simulink model "VSM_specComp_DC_22a"  (R2022a)
settings: Solver=ode3  StartTime=0.0  StopTime=4  FixedStep=HWSampleTime  RelTol=1e-3
PostLoadFcn:
  | EXEC_MODE=ExecutionMode.SIMULATION;
  | %Sim_TP33_VSM_HSS_init
InitFcn:
  | %EXEC_MODE=ExecutionMode.SIMULATION;
  | %Sim_TP33_VSM_HSS_init
StopFcn:
  | %sim2struct
undefined symbols (not defined in the file): ControlSampleTime, DiscIntNeverNeededParam, fault_dur, Grid, HWSampleTime, Ion, LCL, Lithium, Manage, Param, SM, t_fault, V_DC, VSMCTRL
libraries: FriedrichLibrary x76, simulink x32, TriphaseHardwaremodule x24, spsThreePhaseSeriesRLCBranchLib x8, spsThreePhaseVIMeasurementLib x8, spsThreePhaseBreakerLib x8, spsGroundLib x4, spsUniversalBridgeLib x4, spsVoltageMeasurementLib x4, spsEdgeDetectorLib x4, spsMeanLib x4, simulink_extras x4
(part 7 of 10)

== system VSM_specComp_DC_22a/VSM_1/VSM1/VSM/CONTROL/Virtual Circuit1/PT1 ==
  U : Inport  SampleTime=Ts
  tau : Inport  Port=2  SampleTime=Ts
  Reset : Inport  Port=3  SampleTime=Ts
  Delay : Delay  DelayLength=1
  Divide : Product  Inputs=*/
  Gain : Gain  Gain=Ts
  Gain1 : Gain  Gain=K
  Saturation : Saturate  UpperLimit=inf  LowerLimit=Ts
  Sum : Sum  Inputs=|++
  Sum2 : Sum  Inputs=|+-
  Switch : Switch  Criteria=u2 > Threshold  SaturateOnIntegerOverflow=off  InputSameDT=off
  Y : Outport
  wires:
  Reset/1 -> Switch/2
  Saturation/1 -> Divide/2
  Divide/1 -> Sum/1
  tau/1 -> Saturation/1
  Delay/1 -> Sum2/2, Sum/2
  Gain/1 -> Divide/1
  U/1 -> Switch/1, Sum2/1
  Sum2/1 -> Gain/1
  Gain1/1 -> Y/1
  Switch/1 -> Gain1/1, Delay/1
  Sum/1 -> Switch/3

== system VSM_specComp_DC_22a/VSM_1/VSM1/VSM/CONTROL/Virtual Circuit1/PT2 ==
  U : Inport  SampleTime=Ts
  tau : Inport  Port=2  SampleTime=Ts
  Reset : Inport  Port=3  SampleTime=Ts
  Phi : Inport  Port=4
  Delay : Delay  DelayLength=1  InitialConditionSource=Input port  ExternalReset=Rising
      settings: InputPortMap=u0,r5,p4
  Divide : Product  Inputs=*/
  Gain : Gain  Gain=Ts
  Gain1 : Gain  Gain=K
  Saturation : Saturate  UpperLimit=inf  LowerLimit=Ts
  Sum : Sum  Inputs=|++
  Sum2 : Sum  Inputs=|+-
  Unit Delay2 : UnitDelay  InitialCondition=[0 0 0]  SampleTime=ControlSampleTime  HasFrameUpgradeWarning=on
  dq0->ab0 phi1 : FriedrichLibrary/Transformations/dq0->ab0 phi  SystemSampleTime=-1  VariantActivationTime=update diagram  Latency=0  AutoFrameSizeCalculation=off
  Y : Outport
  wires:
  dq0->ab0 phi1/1 -> Delay/3
  Gain1/1 -> Y/1
  Sum2/1 -> Gain/1
  U/1 -> Sum2/1
  Gain/1 -> Divide/1
  Delay/1 -> Sum/2, Sum2/2
  tau/1 -> Saturation/1
  Divide/1 -> Sum/1
  Saturation/1 -> Divide/2
  Reset/1 -> Delay/2
  Sum/1 -> Delay/1, Unit Delay2/1, Gain1/1
  Unit Delay2/1 -> dq0->ab0 phi1/1
  Phi/1 -> dq0->ab0 phi1/2

== system VSM_specComp_DC_22a/VSM_1/VSM1/VSM/CONTROL/i_dq_ctrl/PI ==
  di : Inport
  u0 : Inport  Port=2
  Enable : EnablePort  StatesWhenEnabling=reset
  Gain4 : Gain  Gain=Ki
  Gain5 : Gain  Gain=Kp
  Integrator (inertia) : DiscreteIntegrator  gainval=1  InitialConditionSource=external  InitialCondition=1  SampleTime=ControlSampleTime  ICPrevOutput=DiscIntNeverNeededParam  ICPrevScaledInput=DiscIntNeverNeededParam
  Product : Product
  Product1 : Product
  Step : Step  Time=8  Before=1  SampleTime=0
  Step1 : Step  Time=8.05+10  Before=1  After=0.1  SampleTime=0
  Sum2 : Sum  Inputs=++|
  u : Outport  VectorParamsAs1DForOutWhenUnconnected=off
  wires:
  u0/1 -> Integrator (inertia)/2
  Sum2/1 -> u/1
  di/1 -> Gain4/1, Gain5/1
  Integrator (inertia)/1 -> Sum2/2
  Gain5/1 -> Product/2
  Gain4/1 -> Product1/2
  Product1/1 -> Integrator (inertia)/1
  Product/1 -> Sum2/1
  Step/1 -> Product/1
  Step1/1 -> Product1/1

== system VSM_specComp_DC_22a/VSM_1/VSM1/VSM/MANAGEMENT/Subsystem1/Subsystem ==
  note: zweiter Faktor bei clearing für richtiges Q
      |
      | bei Eintritt mit Halten aber fester Grenze
      |
      | bis jetzt über Zeit abgeschaltet bei clearing ohne Halten
  i_inv : Inport
  PQ_out : Inport  Port=2
  iabs : Inport  Port=3
  U_cap : Inport  Port=4
  PQ_pre : Inport  Port=5
  i abs_pre : Inport  Port=6
  Enable : EnablePort
  Abs : Abs  SaturateOnIntegerOverflow=off
  Add : Sum  Inputs=+-
  Demux : Demux  Commented=on  Outputs=3
  Discrete Derivative1 : simulink/Discrete/Discrete Derivative  Commented=on  gainval=1.0  ICPrevScaledInput=0.0  OutMin=[]  OutMax=[]  OutDataType=fixdt(1, 16)  OutScaling=2^-10  DoSatur=off
  Discrete Derivative2 : simulink/Discrete/Discrete Derivative  gainval=1.0  ICPrevScaledInput=0.0  OutMin=[]  OutMax=[]  OutDataType=fixdt(1, 16)  OutScaling=2^-10  DoSatur=off
  Divide : Product  Inputs=*/
  Divide1 : Product  Commented=on  Inputs=*/
  MATLAB Function1 : MATLAB Function  TreatAsAtomicUnit=on  SystemSampleTime=ControlSampleTime
  MATLAB Function2 : MATLAB Function  Commented=on  TreatAsAtomicUnit=on  SystemSampleTime=ControlSampleTime
  Mean : spsMeanLib/Mean  Freq=2000/2  Vinit=0  Ts=0
  Mux : Mux  Commented=on  Inputs=3
  Rate Transition : RateTransition  Commented=on  OutPortSampleTime=ControlSampleTime
  Scope : Scope  NumInputPorts=2
  Selector1 : Selector  Commented=on  InputPortWidth=3  IndexOptions=Index vector (dialog)  Indices=2  OutputSizes=1
  Selector2 : Selector  InputPortWidth=3  IndexOptions=Index vector (dialog)  Indices=1  OutputSizes=1
  T->ControlSampleTime : Subsystem  Commented=on  TreatAsAtomicUnit=on  SystemSampleTime=ControlSampleTime
  Transfer Fcn : TransferFcn  Commented=on  Denominator=[0.0001 1]
  Transport Delay : TransportDelay  DelayTime=0.002
  i_sp : Outport
  CC : Outport  Port=2
  wires:
  PQ_out/1 -> MATLAB Function1/2(PQ_out)
  iabs/1 -> MATLAB Function1/3(i_abs)
  T->ControlSampleTime/1(Out1) -> Demux/1
  U_cap/1 -> Add/1, Transport Delay/1, Divide1/2, Divide/2, MATLAB Function1/5(U_cap)
  Demux/2 -> Transfer Fcn/1
  Transfer Fcn/1 -> Rate Transition/1
  Demux/1 -> Mux/1
  Demux/3 -> Mux/3
  Rate Transition/1 -> Mux/2
  MATLAB Function1/1(i_sp) -> Scope/1, i_sp/1
  MATLAB Function1/2(CC) -> CC/1
  Selector2/1 -> Divide/1
  Divide/1 -> Discrete Derivative2/1
  PQ_pre/1 -> MATLAB Function1/6(i_pq_pre)
  i abs_pre/1 -> MATLAB Function1/7(i_abs_pre)
  Transport Delay/1 -> Add/2
  Add/1 -> Scope/2, MATLAB Function1/8(u_diff)
  i_inv/1 -> Selector1/1, Selector2/1, T->ControlSampleTime/1(In1), MATLAB Function1/1(i_inv)
  Selector1/1 -> Divide1/1
  Divide1/1 -> Discrete Derivative1/1
  Abs/1 -> Mean/1
  Discrete Derivative2/1 -> Abs/1
  Mean/1 -> MATLAB Function1/4(der)

== system VSM_specComp_DC_22a/VSM_1/VSM1/VSM/MANAGEMENT/Subsystem1/Subsystem1 ==
  In1 : Inport
  In2 : Inport  Port=2
  Enable : EnablePort
  i_pq_pre : Outport
  i_abs_pre : Outport  Port=2
  wires:
  In1/1 -> i_pq_pre/1
  In2/1 -> i_abs_pre/1

== system VSM_specComp_DC_22a/VSM_1/VSM1/VSM/MANAGEMENT/sp_VSM/E(PQ) ==
  E : Inport
  cmd : Inport  Port=2
  sp_PQ : Inport  Port=3
  Abs : Abs  SaturateOnIntegerOverflow=off
  Add : Sum
  Add1 : Sum  Inputs=--
  Add2 : Sum  Inputs=+++
  Bus Selector : BusSelector  OutputSignals=Param.VC.R1,Param.VC.R1t,Param.VC.L1,Param.VC.L1t,Param.VSM.ku
  Bus Selector1 : BusSelector  OutputSignals=Param.VSM.sp_E_comp
  Constant : Constant
  Demux : Demux  Outputs=2
  Display{,1..4} (5 alike) : Display
  Divide : Product  Inputs=/*
  Product : Product
  Product1 : Product
  Real-Imag to Complex : RealImagToComplex
  Real-Imag to Complex1 : RealImagToComplex
  Switch : Switch  Criteria=u2 ~= 0  SaturateOnIntegerOverflow=off  InputSameDT=off
  "cmd " : InportShadow  Port=2
  sp_E : Outport  VectorParamsAs1DForOutWhenUnconnected=off
  wires:
  Add2/1 -> Display3/1, Abs/1
  Abs/1 -> Display4/1, Switch/1
  Product/1 -> Display2/1, Add2/2  "voltage"
  Real-Imag to Complex/1 -> Display1/1, Product/2  "impedance"
  Divide/1 -> Display/1, Product/1  "current"
  Real-Imag to Complex1/1 -> Divide/2
  Demux/2 -> Product1/1, Real-Imag to Complex1/2
  Demux/1 -> Real-Imag to Complex1/1
  sp_PQ/1 -> Demux/1
  E/1 -> Switch/3
  Add1/1 -> Real-Imag to Complex/2
  Add/1 -> Real-Imag to Complex/1
  Bus Selector/4 -> Add1/2  "<L1t>"
  Bus Selector/3 -> Add1/1  "<L1>"
  Bus Selector/2 -> Add/2  "<R1t>"
  Bus Selector/1 -> Add/1  "<R1>"
  cmd/1 -> Bus Selector/1
  Switch/1 -> sp_E/1
  "cmd "/1 -> Bus Selector1/1
  Bus Selector1/1 -> Switch/2  "<sp_E_comp>"
  Bus Selector/5 -> Product1/2  "<ku>"
  Product1/1 -> Add2/3
  Constant/1 -> Divide/1, Add2/1

== system VSM_specComp_DC_22a/VSM_1/VSM1/VSM/MANAGEMENT/sp_VSM/PQ(U) Limit ==
  note: hier muss mit der Leistungsvorgabe multipliziert werden
      | 0.8 U * P0
  sp_PQ : Inport
  enable : Inport  Port=2
  u_out : Inport  Port=3
  Add : Sum
  Constant : Constant
  Dead Zone : DeadZone  LowerValue=0.95  UpperValue=1.05
  Demux : Demux  Outputs=2
  Demux1 : Demux  Outputs=2
  Math Function : Math  Operator=hypot  SignedPower=on
  MinMax : MinMax  Inputs=2
  Mux : Mux  Inputs=2
  Product : Product
  Scope : Scope
  Selector2 : Selector  InputPortWidth=3  IndexOptions=Index vector (dialog)  Indices=[1 2]  OutputSizes=1
  Switch : Switch  Criteria=u2 ~= 0  SaturateOnIntegerOverflow=off  InputSameDT=off
  sp_PQ_limit : Outport  VectorParamsAs1DForOutWhenUnconnected=off
  wires:
  Selector2/1 -> Demux/1
  Demux/1 -> Math Function/1
  Demux/2 -> Math Function/2
  Math Function/1 -> Dead Zone/1
  u_out/1 -> Selector2/1
  sp_PQ/1 -> Switch/3, Demux1/1
  Demux1/2 -> Mux/2
  Demux1/1 -> MinMax/2, Product/2
  MinMax/1 -> Mux/1
  Mux/1 -> Switch/1
  Switch/1 -> Scope/1, sp_PQ_limit/1
  enable/1 -> Switch/2
  Product/1 -> MinMax/1
  Dead Zone/1 -> Add/2
  Add/1 -> Product/1
  Constant/1 -> Add/1

== system VSM_specComp_DC_22a/VSM_1/VSM1/VSM/MANAGEMENT/sp_VSM/RateLimit ==
  PQ : Inport
  Enable : EnablePort
  Compare To Zero : simulink/Logic and Bit Operations/Compare To Zero  relop=>  OutDataTypeStr=boolean
  Constant1 : Constant  Value=Mgn.PQSpRateUp  SampleTime=ControlSampleTime
  Constant2 : Constant  Value=Mgn.PQSpRateDown  SampleTime=ControlSampleTime
  Constant6 : Constant  Value=Mgn.PQSpRateDown  SampleTime=ControlSampleTime
  Constant7 : Constant  Value=Mgn.PQSpRateUp  SampleTime=ControlSampleTime
  Constant8 : Constant  Value=[0 0]  SampleTime=ControlSampleTime
  Logical Operator : Logic  Inputs=1  AllPortsSameDT=off  OutDataTypeStr=boolean
  Mux : Mux  Inputs=2
  Switch : Switch  Criteria=u2 > Threshold  SaturateOnIntegerOverflow=off  InputSameDT=off
  ratelimitspPQ : Subsystem  mask{Ts=ControlSampleTime}
      mask DialogControl ParameterGroupVar Prompt: Rate Limiter
  PQslow : Outport  VectorParamsAs1DForOutWhenUnconnected=off
  wires:
  Logical Operator/1 -> Switch/2
  Mux/1 -> Compare To Zero/1
  Constant2/1 -> Mux/2
  Constant1/1 -> Mux/1
  Compare To Zero/1 -> Logical Operator/1
  Constant7/1 -> ratelimitspPQ/1(rateup)
  Switch/1 -> PQslow/1  "sp_PQ"
  Constant6/1 -> ratelimitspPQ/3(ratedown)
  Constant8/1 -> ratelimitspPQ/4(x0)
  PQ/1 -> ratelimitspPQ/2(x), Switch/1, Switch/3

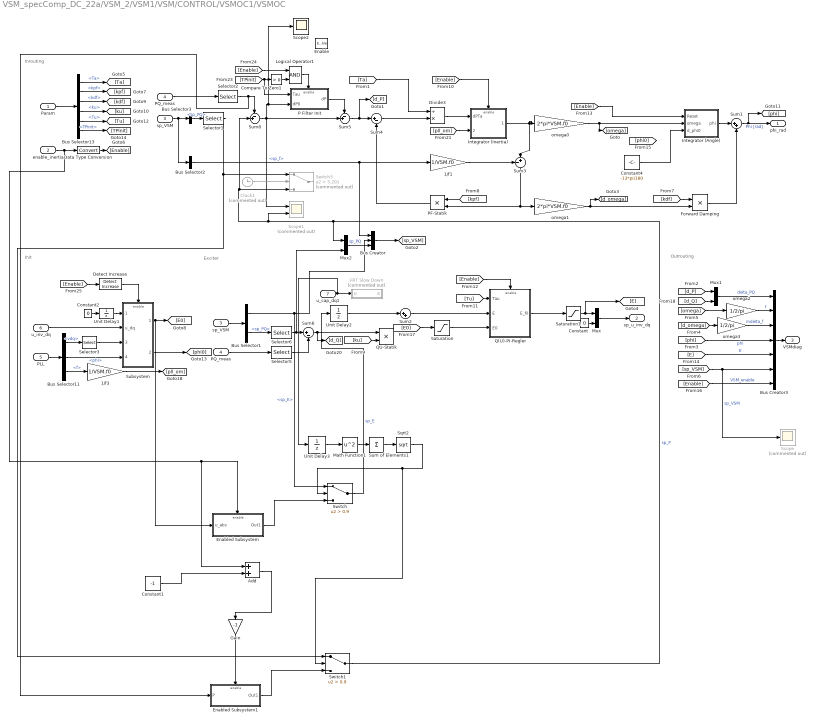
== system VSM_specComp_DC_22a/VSM_2/VSM1/VSM/CONTROL/VSMOC1/VSMOC ==
  note: Inrouting
  note: Exciter
  note: Init
  note: Outrouting
  Param : Inport
  enable_inertia : Inport  Port=2
  sp_VSM : Inport  Port=3
  PQ_meas : Inport  Port=4
  PLL : Inport  Port=5
  u_inv_dq : Inport  Port=6
  u_cap_dq1 : Inport  Port=7
  Enable : EnablePort  StatesWhenEnabling=reset
  1/f1 : Gain  Gain=1/VSM.f0
  1/f3 : Gain  Gain=1/VSM.f0
  Add : Sum
  Bus Creator : BusCreator  Inputs=3
  Bus Creator3 : BusCreator  Inputs=7
  Bus Selector1 : BusSelector  OutputSignals=sp_E,sp_PQ
  Bus Selector11 : BusSelector  OutputSignals=vdq,phi,f
  Bus Selector13 : BusSelector  OutputSignals=Ta,kpf,kdf,ku,Tu,TPinit
  Bus Selector2 : BusSelector  OutputSignals=sp_f
  Bus Selector3 : BusSelector  OutputSignals=sp_PQ
  Clock1 : Clock  Commented=on
  Compare To Zero1 : simulink/Logic and Bit Operations/Compare To Zero  relop=>  OutDataTypeStr=boolean
  Constant : Constant  Value=0
  Constant1 : Constant  Value=-1
  Constant2 : Constant  Value=0  SampleTime=ControlSampleTime
  Constant4 : Constant  Value=-13*pi/180
  Data Type Conversion : DataTypeConversion  SaturateOnIntegerOverflow=off  RndMeth=Floor
  Detect Increase : simulink/Logic and Bit Operations/Detect Increase  vinit=0.0  OutDataTypeStr=boolean
  Divide3 : Product  Inputs=/*
  Enabled Subsystem : Subsystem  TreatAsAtomicUnit=on
  Enabled Subsystem1 : Subsystem  TreatAsAtomicUnit=on
  FRT Slow Down : Subsystem  Commented=on
  Forward Damping : Product  Inputs=**
  Gain : Gain  Gain=-1
  Integrator (Angle) : Subsystem
  Integrator (Inertia) : Subsystem
  Logical Operator1 : Logic  AllPortsSameDT=off  OutDataTypeStr=boolean
  Math Function1 : Math  Operator=square  SignedPower=on
  Mux : Mux  Inputs=2
  Mux1 : Mux  Inputs=2
  Mux2 : Mux  Inputs=2
  P Filter Init : Subsystem
  PF-Statik : Product  Inputs=**
  "PQ_meas " : InportShadow  Port=4
  Q(U)-PI-Regler : Subsystem
  QU-Statik : Product  Inputs=**
  Saturation : Saturate  UpperLimit=1.8  LowerLimit=0.8*0
  Saturation1 : Saturate  UpperLimit=2
  Scope : Scope  Commented=on
  Scope1 : Scope  Commented=on  NumInputPorts=2
  Scope2 : Scope
  Selector1 : Selector  InputPortWidth=2  IndexOptions=Index vector (dialog)  Indices=1  OutputSizes=1
  Selector2 : Selector  InputPortWidth=2  IndexOptions=Index vector (dialog)  Indices=1  OutputSizes=1
  Selector3 : Selector  InputPortWidth=3  IndexOptions=Index vector (dialog)  Indices=[1 2]  OutputSizes=1
  Selector5 : Selector  InputPortWidth=2  IndexOptions=Index vector (dialog)  Indices=2  OutputSizes=1
  Selector6 : Selector  InputPortWidth=2  IndexOptions=Index vector (dialog)  Indices=2  OutputSizes=1
  Sqrt2 : Sqrt
  Subsystem : Subsystem
  Sum of Elements1 : Sum  Inputs=+
  Sum1 : Sum  Inputs=|++
  Sum2 : Sum  Inputs=|++
  Sum3 : Sum  Inputs=-+|
  Sum4 : Sum  Inputs=|+-
  Sum5 : Sum  Inputs=-+|
  Sum6 : Sum  Inputs=|+-
  Sum8 : Sum  Inputs=-+|
  Switch : Switch  Criteria=u2 > Threshold  Threshold=0.9  SaturateOnIntegerOverflow=off  InputSameDT=off
  Switch1 : Switch  Criteria=u2 > Threshold  Threshold=0.9  SaturateOnIntegerOverflow=off  InputSameDT=off
  Switch3 : Switch  Commented=on  Criteria=u2 > Threshold  Threshold=5.201  SaturateOnIntegerOverflow=off  InputSameDT=off
  Unit Delay1 : UnitDelay  InitialCondition=1  SampleTime=ControlSampleTime  HasFrameUpgradeWarning=on
  Unit Delay2 : UnitDelay  SampleTime=-1  HasFrameUpgradeWarning=on
  Unit Delay3 : UnitDelay  SampleTime=-1  HasFrameUpgradeWarning=on
  omega0 : Gain  Gain=2*pi*VSM.f0
  omega1 : Gain  Gain=2*pi*VSM.f0
  omega2 : Gain  Gain=1/2/pi
  omega3 : Gain  Gain=1/2/pi
  "sp_VSM " : InportShadow  Port=3
  phi_rad : Outport  VectorParamsAs1DForOutWhenUnconnected=off
  sp_u_inv_dq : Outport  Port=2  InitialOutput=[1 0]  VectorParamsAs1DForOutWhenUnconnected=off
  VSMdiag : Outport  Port=3  VectorParamsAs1DForOutWhenUnconnected=off
  wires:
  [Enable] -> Q(U)-PI-Regler/Enable
  Bus Selector11/2 -> Subsystem/4(phi_pll)  "<phi>"
  Selector5/1 -> Sum6/2
  Selector6/1 -> Mux2/2, Sum6/1
  1/f1/1 -> Sum3/1
  [d_Q] -> Mux1/2
  [d_P] -> Mux1/1
  Mux1/1 -> Bus Creator3/1  "delta_PQ"
  Selector2/1 -> Enabled Subsystem1/1(P), Sum8/1
  Sum6/1 -> QU-Statik/1, [d_Q]
  "sp_VSM "/1 -> Bus Selector1/1
  Bus Selector1/2 -> Selector6/1  "<sp_PQ>"
  "PQ_meas "/1 -> Selector5/1
  [kpf] -> PF-Statik/1
  [kdf] -> Forward Damping/1
  1/f3/1 -> [pll_om]
  Bus Selector11/3 -> 1/f3/1  "<f>"
  Integrator (Angle)/1(phi) -> Sum1/1
  Selector3/1 -> Subsystem/3(u_dq_pll)
  [Enable] -> Bus Creator3/7  "VSM_enable"
  Sum1/1 -> [phi], phi_rad/1  "Phi [rad]"
  Sum4/1 -> Divide3/2
  Sum3/1 -> PF-Statik/2, omega1/1
  Bus Selector2/1 -> Bus Creator/1, 1/f1/1  "<sp_f>"
  PLL/1 -> Bus Selector11/1
  Bus Creator3/1 -> VSMdiag/1
  [omega] -> omega2/1
  omega1/1 -> Forward Damping/2, [d_omega]
  [d_omega] -> omega3/1
  omega2/1 -> Bus Creator3/2  "f"
  omega3/1 -> Bus Creator3/3  "mdelta_f"
  [sp_VSM] -> Scope/1, Bus Creator3/6  "sp_VSM"
  PQ_meas/1 -> Selector2/1
  Bus Selector11/1 -> Selector3/1  "<vdq>"
  Divide3/1 -> Integrator (Inertia)/1(dPTa)
  [pll_om] -> Integrator (Inertia)/2(omega0 [pu])
  Mux/1 -> sp_u_inv_dq/1
  Constant/1 -> Mux/2
  Subsystem/2(u_ang) -> [phi0]
  Detect Increase/1 -> Subsystem/Enable
  Sum5/1 -> Sum4/1, [d_P]
  [TPinit] -> P Filter Init/1(Tau), Compare To Zero1/1
  Compare To Zero1/1 -> Logical Operator1/2
  Logical Operator1/1 -> P Filter Init/Enable
  [Enable] -> Logical Operator1/1
  Bus Selector13/5 -> [Tu]  "<Tu>"
  Bus Selector13/4 -> [ku]  "<ku>"
  Bus Selector13/3 -> [kdf]  "<kdf>"
  Bus Selector13/2 -> [kpf]  "<kpf>"
  Bus Selector13/1 -> [Ta]  "<Ta>"
  Param/1 -> Bus Selector13/1
  [Enable] -> Detect Increase/1
  u_inv_dq/1 -> Subsystem/2(u_dq)
  Constant2/1 -> Unit Delay1/1
  Unit Delay1/1 -> Subsystem/1(first_run)
  Data Type Conversion/1 -> [Enable]
  Sum2/1 -> Q(U)-PI-Regler/2(E)
  [ku] -> QU-Statik/2
  [E] -> Bus Creator3/5  "E"
  Bus Selector13/6 -> [TPinit]  "<TPinit>"
  [phi] -> Bus Creator3/4  "phi"
  [Tu] -> Q(U)-PI-Regler/1(Tau)
  Unit Delay2/1 -> Sum2/1
  [E0] -> Saturation/1
  [Enable] -> Integrator (Angle)/1(Reset)
  omega0/1 -> Integrator (Angle)/2(omega), [omega]
  Saturation1/1 -> [E], Mux/1
  Forward Damping/1 -> Sum1/2
  [Enable] -> Integrator (Inertia)/Enable
  Integrator (Inertia)/1(omega [pu]) -> omega0/1, Sum3/2
  Bus Selector3/1 -> Selector1/1  "<sp_PQ>"
  sp_VSM/1 -> Bus Selector2/1, Bus Selector3/1
  Sum8/1 -> Scope1/1, Sum5/2, Scope2/1, P Filter Init/2(dP0)
  [Ta] -> Divide3/1
  P Filter Init/1(dP) -> Sum5/1
  PF-Statik/1 -> Sum4/2
  Sqrt2/1 -> Switch1/2, Switch/2
  u_cap_dq1/1 -> Unit Delay3/1, FRT Slow Down/1(U)
  Sum of Elements1/1 -> Sqrt2/1
  Unit Delay3/1 -> Math Function1/1
  Math Function1/1 -> Sum of Elements1/1
  Bus Selector1/1 -> Bus Creator/2, Switch/1  "<sp_E>"
  enable_inertia/1 -> Add/1, Enabled Subsystem/Enable, Data Type Conversion/1
  Enabled Subsystem/1(Out1) -> Switch/3
  Subsystem/1(u_abs) -> Enabled Subsystem/1(u_abs), [E0]
  Enabled Subsystem1/1(Out1) -> Switch1/3
  Switch/1 -> Unit Delay2/1  "sp_E"
  Switch1/1 -> Scope1/2, Sum8/2, Switch3/3, Mux2/1  "sp_P"
  Clock1/1 -> Switch3/2
  Q(U)-PI-Regler/1(E_fil) -> Saturation1/1
  Selector1/1 -> Switch3/1, Switch1/1
  Constant1/1 -> Add/2
  Gain/1 -> Enabled Subsystem1/Enable
  Add/1 -> Gain/1
  Mux2/1 -> Bus Creator/3  "sp_PQ"
  Bus Creator/1 -> [sp_VSM]
  Constant4/1 -> Integrator (Angle)/3(d_phi0)
  Saturation/1 -> Q(U)-PI-Regler/3(E0)

== system VSM_specComp_DC_22a/VSM_2/VSM1/VSM/CONTROL/Virtual Circuit mit R und L/Current Predictor ==
  u : Inport
  Delay : Delay  DelayLength=1  InitialCondition=0
  Sum : Sum  Inputs=|-+
  Sum1 : Sum  Inputs=|++
  y : Outport
  wires:
  u/1 -> Sum/2, Sum1/2, Delay/1
  Delay/1 -> Sum/1
  Sum/1 -> Sum1/1
  Sum1/1 -> y/1

== system VSM_specComp_DC_22a/VSM_2/VSM1/VSM/CONTROL/Virtual Circuit mit R und L/PT1 ==
  U : Inport  SampleTime=Ts
  tau : Inport  Port=2  SampleTime=Ts
  Reset : Inport  Port=3  SampleTime=Ts
  Phi : Inport  Port=4
  Delay : Delay  DelayLength=1  InitialConditionSource=Input port  ExternalReset=Rising
      settings: InputPortMap=u0,r5,p4
  Divide : Product  Inputs=*/
  Gain : Gain  Gain=Ts
  Gain1 : Gain  Gain=K
  Saturation : Saturate  UpperLimit=inf  LowerLimit=Ts
  Sum : Sum  Inputs=|++
  Sum2 : Sum  Inputs=|+-
  Unit Delay2 : UnitDelay  InitialCondition=[0 0 0]  SampleTime=ControlSampleTime  HasFrameUpgradeWarning=on
  dq0->ab0 phi : FriedrichLibrary/Transformations/dq0->ab0 phi  SystemSampleTime=-1  VariantActivationTime=update diagram  Latency=0  AutoFrameSizeCalculation=off
  Y : Outport
  wires:
  Phi/1 -> dq0->ab0 phi/2
  Unit Delay2/1 -> dq0->ab0 phi/1
  Sum/1 -> Gain1/1, Unit Delay2/1, Delay/1
  Reset/1 -> Delay/2
  Saturation/1 -> Divide/2
  Divide/1 -> Sum/1
  tau/1 -> Saturation/1
  Delay/1 -> Sum2/2, Sum/2
  Gain/1 -> Divide/1
  U/1 -> Sum2/1
  Sum2/1 -> Gain/1
  Gain1/1 -> Y/1
  dq0->ab0 phi/1 -> Delay/3

== system VSM_specComp_DC_22a/VSM_2/VSM1/VSM/CONTROL/Virtual Circuit mit R und L/PT2 ==
  U : Inport  SampleTime=Ts
  tau : Inport  Port=2  SampleTime=Ts
  Reset : Inport  Port=3  SampleTime=Ts
  Phi : Inport  Port=4
  Delay : Delay  DelayLength=1  InitialConditionSource=Input port  ExternalReset=Rising
      settings: InputPortMap=u0,r5,p4
  Divide : Product  Inputs=*/
  Gain : Gain  Gain=Ts
  Gain1 : Gain  Gain=K
  Saturation : Saturate  UpperLimit=inf  LowerLimit=Ts
  Sum : Sum  Inputs=|++
  Sum2 : Sum  Inputs=|+-
  Unit Delay2 : UnitDelay  InitialCondition=[0 0 0]  SampleTime=ControlSampleTime  HasFrameUpgradeWarning=on
  dq0->ab0 phi1 : FriedrichLibrary/Transformations/dq0->ab0 phi  SystemSampleTime=-1  VariantActivationTime=update diagram  Latency=0  AutoFrameSizeCalculation=off
  Y : Outport
  wires:
  dq0->ab0 phi1/1 -> Delay/3
  Gain1/1 -> Y/1
  Sum2/1 -> Gain/1
  U/1 -> Sum2/1
  Gain/1 -> Divide/1
  Delay/1 -> Sum/2, Sum2/2
  tau/1 -> Saturation/1
  Divide/1 -> Sum/1
  Saturation/1 -> Divide/2
  Reset/1 -> Delay/2
  Sum/1 -> Delay/1, Unit Delay2/1, Gain1/1
  Unit Delay2/1 -> dq0->ab0 phi1/1
  Phi/1 -> dq0->ab0 phi1/2

== system VSM_specComp_DC_22a/VSM_2/VSM1/VSM/CONTROL/Virtual Circuit1/Current Predictor ==
  u : Inport
  Delay : Delay  DelayLength=1  InitialCondition=0
  Sum : Sum  Inputs=|-+
  Sum1 : Sum  Inputs=|++
  y : Outport
  wires:
  u/1 -> Sum/2, Sum1/2, Delay/1
  Delay/1 -> Sum/1
  Sum/1 -> Sum1/1
  Sum1/1 -> y/1

== system VSM_specComp_DC_22a/VSM_2/VSM1/VSM/CONTROL/Virtual Circuit1/PT1 ==
  U : Inport  SampleTime=Ts
  tau : Inport  Port=2  SampleTime=Ts
  Reset : Inport  Port=3  SampleTime=Ts
  Delay : Delay  DelayLength=1
  Divide : Product  Inputs=*/
  Gain : Gain  Gain=Ts
  Gain1 : Gain  Gain=K
  Saturation : Saturate  UpperLimit=inf  LowerLimit=Ts
  Sum : Sum  Inputs=|++
  Sum2 : Sum  Inputs=|+-
  Switch : Switch  Criteria=u2 > Threshold  SaturateOnIntegerOverflow=off  InputSameDT=off
  Y : Outport
  wires:
  Reset/1 -> Switch/2
  Saturation/1 -> Divide/2
  Divide/1 -> Sum/1
  tau/1 -> Saturation/1
  Delay/1 -> Sum2/2, Sum/2
  Gain/1 -> Divide/1
  U/1 -> Switch/1, Sum2/1
  Sum2/1 -> Gain/1
  Gain1/1 -> Y/1
  Switch/1 -> Gain1/1, Delay/1
  Sum/1 -> Switch/3

== system VSM_specComp_DC_22a/VSM_2/VSM1/VSM/CONTROL/Virtual Circuit1/PT2 ==
  U : Inport  SampleTime=Ts
  tau : Inport  Port=2  SampleTime=Ts
  Reset : Inport  Port=3  SampleTime=Ts
  Phi : Inport  Port=4
  Delay : Delay  DelayLength=1  InitialConditionSource=Input port  ExternalReset=Rising
      settings: InputPortMap=u0,r5,p4
  Divide : Product  Inputs=*/
  Gain : Gain  Gain=Ts
  Gain1 : Gain  Gain=K
  Saturation : Saturate  UpperLimit=inf  LowerLimit=Ts
  Sum : Sum  Inputs=|++
  Sum2 : Sum  Inputs=|+-
  Unit Delay2 : UnitDelay  InitialCondition=[0 0 0]  SampleTime=ControlSampleTime  HasFrameUpgradeWarning=on
  dq0->ab0 phi1 : FriedrichLibrary/Transformations/dq0->ab0 phi  SystemSampleTime=-1  VariantActivationTime=update diagram  Latency=0  AutoFrameSizeCalculation=off
  Y : Outport
  wires:
  dq0->ab0 phi1/1 -> Delay/3
  Gain1/1 -> Y/1
  Sum2/1 -> Gain/1
  U/1 -> Sum2/1
  Gain/1 -> Divide/1
  Delay/1 -> Sum/2, Sum2/2
  tau/1 -> Saturation/1
  Divide/1 -> Sum/1
  Saturation/1 -> Divide/2
  Reset/1 -> Delay/2
  Sum/1 -> Delay/1, Unit Delay2/1, Gain1/1
  Unit Delay2/1 -> dq0->ab0 phi1/1
  Phi/1 -> dq0->ab0 phi1/2

== system VSM_specComp_DC_22a/VSM_2/VSM1/VSM/CONTROL/i_dq_ctrl/PI ==
  di : Inport
  u0 : Inport  Port=2
  Enable : EnablePort  StatesWhenEnabling=reset
  Gain4 : Gain  Gain=Ki
  Gain5 : Gain  Gain=Kp
  Integrator (inertia) : DiscreteIntegrator  gainval=1  InitialConditionSource=external  InitialCondition=1  SampleTime=ControlSampleTime  ICPrevOutput=DiscIntNeverNeededParam  ICPrevScaledInput=DiscIntNeverNeededParam
  Product : Product
  Product1 : Product
  Step : Step  Time=8  Before=1  SampleTime=0
  Step1 : Step  Time=8.05+10  Before=1  After=0.1  SampleTime=0
  Sum2 : Sum  Inputs=++|
  u : Outport  VectorParamsAs1DForOutWhenUnconnected=off
  wires:
  u0/1 -> Integrator (inertia)/2
  Sum2/1 -> u/1
  di/1 -> Gain4/1, Gain5/1
  Integrator (inertia)/1 -> Sum2/2
  Gain5/1 -> Product/2
  Gain4/1 -> Product1/2
  Product1/1 -> Integrator (inertia)/1
  Product/1 -> Sum2/1
  Step/1 -> Product/1
  Step1/1 -> Product1/1

== system VSM_specComp_DC_22a/VSM_2/VSM1/VSM/MANAGEMENT/Subsystem1/Subsystem ==
  note: zweiter Faktor bei clearing für richtiges Q
      |
      | bei Eintritt mit Halten aber fester Grenze
      |
      | bis jetzt über Zeit abgeschaltet bei clearing ohne Halten
  i_inv : Inport
  PQ_out : Inport  Port=2
  iabs : Inport  Port=3
  U_cap : Inport  Port=4
  PQ_pre : Inport  Port=5
  i abs_pre : Inport  Port=6
  Enable : EnablePort
  Abs : Abs  SaturateOnIntegerOverflow=off
  Add : Sum  Inputs=+-
  Demux : Demux  Commented=on  Outputs=3
  Discrete Derivative1 : simulink/Discrete/Discrete Derivative  Commented=on  gainval=1.0  ICPrevScaledInput=0.0  OutMin=[]  OutMax=[]  OutDataType=fixdt(1, 16)  OutScaling=2^-10  DoSatur=off
  Discrete Derivative2 : simulink/Discrete/Discrete Derivative  gainval=1.0  ICPrevScaledInput=0.0  OutMin=[]  OutMax=[]  OutDataType=fixdt(1, 16)  OutScaling=2^-10  DoSatur=off
  Divide : Product  Inputs=*/
  Divide1 : Product  Commented=on  Inputs=*/
  MATLAB Function1 : MATLAB Function  TreatAsAtomicUnit=on  SystemSampleTime=ControlSampleTime
  MATLAB Function2 : MATLAB Function  Commented=on  TreatAsAtomicUnit=on  SystemSampleTime=ControlSampleTime
  Mean : spsMeanLib/Mean  Freq=2000/2  Vinit=0  Ts=0
  Mux : Mux  Commented=on  Inputs=3
  Rate Transition : RateTransition  Commented=on  OutPortSampleTime=ControlSampleTime
  Scope : Scope  NumInputPorts=2
  Selector1 : Selector  Commented=on  InputPortWidth=3  IndexOptions=Index vector (dialog)  Indices=2  OutputSizes=1
  Selector2 : Selector  InputPortWidth=3  IndexOptions=Index vector (dialog)  Indices=1  OutputSizes=1
  T->ControlSampleTime : Subsystem  Commented=on  TreatAsAtomicUnit=on  SystemSampleTime=ControlSampleTime
  Transfer Fcn : TransferFcn  Commented=on  Denominator=[0.0001 1]
  Transport Delay : TransportDelay  DelayTime=0.002
  i_sp : Outport
  CC : Outport  Port=2
  wires:
  PQ_out/1 -> MATLAB Function1/2(PQ_out)
  iabs/1 -> MATLAB Function1/3(i_abs)
  T->ControlSampleTime/1(Out1) -> Demux/1
  U_cap/1 -> Add/1, Transport Delay/1, Divide1/2, Divide/2, MATLAB Function1/5(U_cap)
  Demux/2 -> Transfer Fcn/1
  Transfer Fcn/1 -> Rate Transition/1
  Demux/1 -> Mux/1
  Demux/3 -> Mux/3
  Rate Transition/1 -> Mux/2
  MATLAB Function1/1(i_sp) -> Scope/1, i_sp/1
  MATLAB Function1/2(CC) -> CC/1
  Selector2/1 -> Divide/1
  Divide/1 -> Discrete Derivative2/1
  PQ_pre/1 -> MATLAB Function1/6(i_pq_pre)
  i abs_pre/1 -> MATLAB Function1/7(i_abs_pre)
  Transport Delay/1 -> Add/2
  Add/1 -> Scope/2, MATLAB Function1/8(u_diff)
  i_inv/1 -> Selector1/1, Selector2/1, T->ControlSampleTime/1(In1), MATLAB Function1/1(i_inv)
  Selector1/1 -> Divide1/1
  Divide1/1 -> Discrete Derivative1/1
  Abs/1 -> Mean/1
  Discrete Derivative2/1 -> Abs/1
  Mean/1 -> MATLAB Function1/4(der)

== system VSM_specComp_DC_22a/VSM_2/VSM1/VSM/MANAGEMENT/Subsystem1/Subsystem1 ==
  In1 : Inport
  In2 : Inport  Port=2
  Enable : EnablePort
  i_pq_pre : Outport
  i_abs_pre : Outport  Port=2
  wires:
  In1/1 -> i_pq_pre/1
  In2/1 -> i_abs_pre/1

== system VSM_specComp_DC_22a/VSM_2/VSM1/VSM/MANAGEMENT/sp_VSM/E(PQ) ==
  E : Inport
  cmd : Inport  Port=2
  sp_PQ : Inport  Port=3
  Abs : Abs  SaturateOnIntegerOverflow=off
  Add : Sum
  Add1 : Sum  Inputs=--
  Add2 : Sum  Inputs=+++
  Bus Selector : BusSelector  OutputSignals=Param.VC.R1,Param.VC.R1t,Param.VC.L1,Param.VC.L1t,Param.VSM.ku
  Bus Selector1 : BusSelector  OutputSignals=Param.VSM.sp_E_comp
  Constant : Constant
  Demux : Demux  Outputs=2
  Display{,1..4} (5 alike) : Display
  Divide : Product  Inputs=/*
  Product : Product
  Product1 : Product
  Real-Imag to Complex : RealImagToComplex
  Real-Imag to Complex1 : RealImagToComplex
  Switch : Switch  Criteria=u2 ~= 0  SaturateOnIntegerOverflow=off  InputSameDT=off
  "cmd " : InportShadow  Port=2
  sp_E : Outport  VectorParamsAs1DForOutWhenUnconnected=off
  wires:
  Add2/1 -> Display3/1, Abs/1
  Abs/1 -> Display4/1, Switch/1
  Product/1 -> Display2/1, Add2/2  "voltage"
  Real-Imag to Complex/1 -> Display1/1, Product/2  "impedance"
  Divide/1 -> Display/1, Product/1  "current"
  Real-Imag to Complex1/1 -> Divide/2
  Demux/2 -> Product1/1, Real-Imag to Complex1/2
  Demux/1 -> Real-Imag to Complex1/1
  sp_PQ/1 -> Demux/1
  E/1 -> Switch/3
  Add1/1 -> Real-Imag to Complex/2
  Add/1 -> Real-Imag to Complex/1
  Bus Selector/4 -> Add1/2  "<L1t>"
  Bus Selector/3 -> Add1/1  "<L1>"
  Bus Selector/2 -> Add/2  "<R1t>"
  Bus Selector/1 -> Add/1  "<R1>"
  cmd/1 -> Bus Selector/1
  Switch/1 -> sp_E/1
  "cmd "/1 -> Bus Selector1/1
  Bus Selector1/1 -> Switch/2  "<sp_E_comp>"
  Bus Selector/5 -> Product1/2  "<ku>"
  Product1/1 -> Add2/3
  Constant/1 -> Divide/1, Add2/1

== system VSM_specComp_DC_22a/VSM_2/VSM1/VSM/MANAGEMENT/sp_VSM/PQ(U) Limit ==
  note: hier muss mit der Leistungsvorgabe multipliziert werden
      | 0.8 U * P0
  sp_PQ : Inport
  enable : Inport  Port=2
  u_out : Inport  Port=3
  Add : Sum
  Constant : Constant
  Dead Zone : DeadZone  LowerValue=0.95  UpperValue=1.05
  Demux : Demux  Outputs=2
  Demux1 : Demux  Outputs=2
  Math Function : Math  Operator=hypot  SignedPower=on
  MinMax : MinMax  Inputs=2
  Mux : Mux  Inputs=2
  Product : Product
  Scope : Scope
  Selector2 : Selector  InputPortWidth=3  IndexOptions=Index vector (dialog)  Indices=[1 2]  OutputSizes=1
  Switch : Switch  Criteria=u2 ~= 0  SaturateOnIntegerOverflow=off  InputSameDT=off
  sp_PQ_limit : Outport  VectorParamsAs1DForOutWhenUnconnected=off
  wires:
  Selector2/1 -> Demux/1
  Demux/1 -> Math Function/1
  Demux/2 -> Math Function/2
  Math Function/1 -> Dead Zone/1
  u_out/1 -> Selector2/1
  sp_PQ/1 -> Switch/3, Demux1/1
  Demux1/2 -> Mux/2
  Demux1/1 -> MinMax/2, Product/2
  MinMax/1 -> Mux/1
  Mux/1 -> Switch/1
  Switch/1 -> Scope/1, sp_PQ_limit/1
  enable/1 -> Switch/2
  Product/1 -> MinMax/1
  Dead Zone/1 -> Add/2
  Add/1 -> Product/1
  Constant/1 -> Add/1

== system VSM_specComp_DC_22a/VSM_2/VSM1/VSM/MANAGEMENT/sp_VSM/RateLimit ==
  PQ : Inport
  Enable : EnablePort
  Compare To Zero : simulink/Logic and Bit Operations/Compare To Zero  relop=>  OutDataTypeStr=boolean
  Constant1 : Constant  Value=Mgn.PQSpRateUp  SampleTime=ControlSampleTime
  Constant2 : Constant  Value=Mgn.PQSpRateDown  SampleTime=ControlSampleTime
  Constant6 : Constant  Value=Mgn.PQSpRateDown  SampleTime=ControlSampleTime
  Constant7 : Constant  Value=Mgn.PQSpRateUp  SampleTime=ControlSampleTime
  Constant8 : Constant  Value=[0 0]  SampleTime=ControlSampleTime
  Logical Operator : Logic  Inputs=1  AllPortsSameDT=off  OutDataTypeStr=boolean
  Mux : Mux  Inputs=2
  Switch : Switch  Criteria=u2 > Threshold  SaturateOnIntegerOverflow=off  InputSameDT=off
  ratelimitspPQ : Subsystem  mask{Ts=ControlSampleTime}
      mask DialogControl ParameterGroupVar Prompt: Rate Limiter
  PQslow : Outport  VectorParamsAs1DForOutWhenUnconnected=off
  wires:
  Logical Operator/1 -> Switch/2
  Mux/1 -> Compare To Zero/1
  Constant2/1 -> Mux/2
  Constant1/1 -> Mux/1
  Compare To Zero/1 -> Logical Operator/1
  Constant7/1 -> ratelimitspPQ/1(rateup)
  Switch/1 -> PQslow/1  "sp_PQ"
  Constant6/1 -> ratelimitspPQ/3(ratedown)
  Constant8/1 -> ratelimitspPQ/4(x0)
  PQ/1 -> ratelimitspPQ/2(x), Switch/1, Switch/3

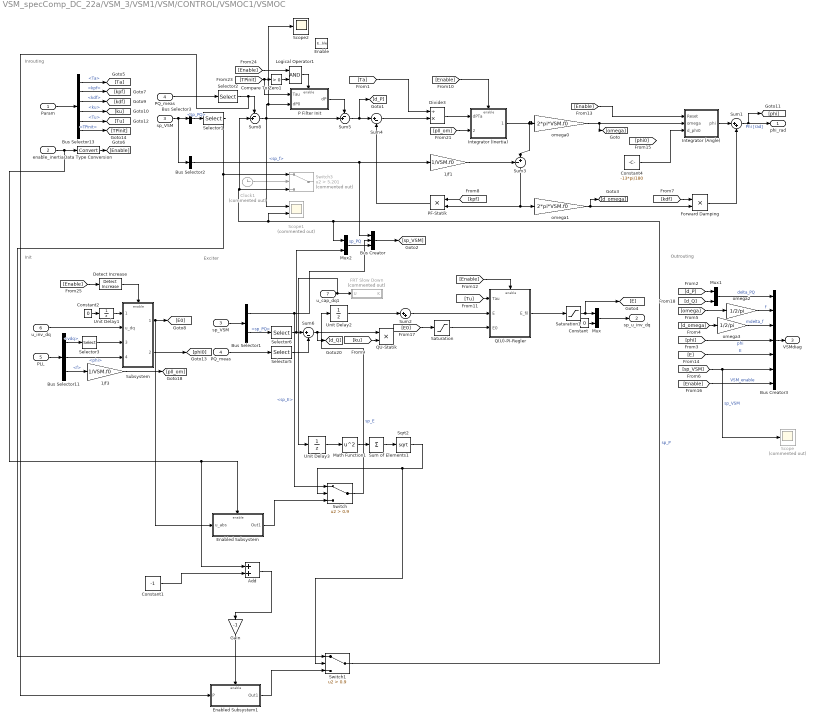
== system VSM_specComp_DC_22a/VSM_3/VSM1/VSM/CONTROL/VSMOC1/VSMOC ==
  note: Outrouting
  note: Init
  note: Exciter
  note: Inrouting
  Param : Inport
  enable_inertia : Inport  Port=2
  sp_VSM : Inport  Port=3
  PQ_meas : Inport  Port=4
  PLL : Inport  Port=5
  u_inv_dq : Inport  Port=6
  u_cap_dq1 : Inport  Port=7
  Enable : EnablePort  StatesWhenEnabling=reset
  1/f1 : Gain  Gain=1/VSM.f0
  1/f3 : Gain  Gain=1/VSM.f0
  Add : Sum
  Bus Creator : BusCreator  Inputs=3
  Bus Creator3 : BusCreator  Inputs=7
  Bus Selector1 : BusSelector  OutputSignals=sp_E,sp_PQ
  Bus Selector11 : BusSelector  OutputSignals=vdq,phi,f
  Bus Selector13 : BusSelector  OutputSignals=Ta,kpf,kdf,ku,Tu,TPinit
  Bus Selector2 : BusSelector  OutputSignals=sp_f
  Bus Selector3 : BusSelector  OutputSignals=sp_PQ
  Clock1 : Clock  Commented=on
  Compare To Zero1 : simulink/Logic and Bit Operations/Compare To Zero  relop=>  OutDataTypeStr=boolean
  Constant : Constant  Value=0
  Constant1 : Constant  Value=-1
  Constant2 : Constant  Value=0  SampleTime=ControlSampleTime
  Constant4 : Constant  Value=-13*pi/180
  Data Type Conversion : DataTypeConversion  SaturateOnIntegerOverflow=off  RndMeth=Floor
  Detect Increase : simulink/Logic and Bit Operations/Detect Increase  vinit=0.0  OutDataTypeStr=boolean
  Divide3 : Product  Inputs=/*
  Enabled Subsystem : Subsystem  TreatAsAtomicUnit=on
  Enabled Subsystem1 : Subsystem  TreatAsAtomicUnit=on
  FRT Slow Down : Subsystem  Commented=on
  Forward Damping : Product  Inputs=**
  Gain : Gain  Gain=-1
  Integrator (Angle) : Subsystem
  Integrator (Inertia) : Subsystem
  Logical Operator1 : Logic  AllPortsSameDT=off  OutDataTypeStr=boolean
  Math Function1 : Math  Operator=square  SignedPower=on
  Mux : Mux  Inputs=2
  Mux1 : Mux  Inputs=2
  Mux2 : Mux  Inputs=2
  P Filter Init : Subsystem
  PF-Statik : Product  Inputs=**
  "PQ_meas " : InportShadow  Port=4
  Q(U)-PI-Regler : Subsystem
  QU-Statik : Product  Inputs=**
  Saturation : Saturate  UpperLimit=1.8  LowerLimit=0.8*0
  Saturation1 : Saturate  UpperLimit=2
  Scope : Scope  Commented=on
  Scope1 : Scope  Commented=on  NumInputPorts=2
  Scope2 : Scope
  Selector1 : Selector  InputPortWidth=2  IndexOptions=Index vector (dialog)  Indices=1  OutputSizes=1
  Selector2 : Selector  InputPortWidth=2  IndexOptions=Index vector (dialog)  Indices=1  OutputSizes=1
  Selector3 : Selector  InputPortWidth=3  IndexOptions=Index vector (dialog)  Indices=[1 2]  OutputSizes=1
  Selector5 : Selector  InputPortWidth=2  IndexOptions=Index vector (dialog)  Indices=2  OutputSizes=1
  Selector6 : Selector  InputPortWidth=2  IndexOptions=Index vector (dialog)  Indices=2  OutputSizes=1
  Sqrt2 : Sqrt
  Subsystem : Subsystem
  Sum of Elements1 : Sum  Inputs=+
  Sum1 : Sum  Inputs=|++
  Sum2 : Sum  Inputs=|++
  Sum3 : Sum  Inputs=-+|
  Sum4 : Sum  Inputs=|+-
  Sum5 : Sum  Inputs=-+|
  Sum6 : Sum  Inputs=|+-
  Sum8 : Sum  Inputs=-+|
  Switch : Switch  Criteria=u2 > Threshold  Threshold=0.9  SaturateOnIntegerOverflow=off  InputSameDT=off
  Switch1 : Switch  Criteria=u2 > Threshold  Threshold=0.9  SaturateOnIntegerOverflow=off  InputSameDT=off
  Switch3 : Switch  Commented=on  Criteria=u2 > Threshold  Threshold=5.201  SaturateOnIntegerOverflow=off  InputSameDT=off
  Unit Delay1 : UnitDelay  InitialCondition=1  SampleTime=ControlSampleTime  HasFrameUpgradeWarning=on
  Unit Delay2 : UnitDelay  SampleTime=-1  HasFrameUpgradeWarning=on
  Unit Delay3 : UnitDelay  SampleTime=-1  HasFrameUpgradeWarning=on
  omega0 : Gain  Gain=2*pi*VSM.f0
  omega1 : Gain  Gain=2*pi*VSM.f0
  omega2 : Gain  Gain=1/2/pi
  omega3 : Gain  Gain=1/2/pi
  "sp_VSM " : InportShadow  Port=3
  phi_rad : Outport  VectorParamsAs1DForOutWhenUnconnected=off
  sp_u_inv_dq : Outport  Port=2  InitialOutput=[1 0]  VectorParamsAs1DForOutWhenUnconnected=off
  VSMdiag : Outport  Port=3  VectorParamsAs1DForOutWhenUnconnected=off
  wires:
  Saturation/1 -> Q(U)-PI-Regler/3(E0)
  Constant4/1 -> Integrator (Angle)/3(d_phi0)
  Bus Creator/1 -> [sp_VSM]
  Mux2/1 -> Bus Creator/3  "sp_PQ"
  Add/1 -> Gain/1
  Gain/1 -> Enabled Subsystem1/Enable
  Constant1/1 -> Add/2
  Selector1/1 -> Switch1/1, Switch3/1
  Q(U)-PI-Regler/1(E_fil) -> Saturation1/1
  Clock1/1 -> Switch3/2
  Switch1/1 -> Mux2/1, Switch3/3, Sum8/2, Scope1/2  "sp_P"
  Switch/1 -> Unit Delay2/1  "sp_E"
  Enabled Subsystem1/1(Out1) -> Switch1/3
  Subsystem/1(u_abs) -> [E0], Enabled Subsystem/1(u_abs)
  Enabled Subsystem/1(Out1) -> Switch/3
  enable_inertia/1 -> Data Type Conversion/1, Enabled Subsystem/Enable, Add/1
  Bus Selector1/1 -> Switch/1, Bus Creator/2  "<sp_E>"
  Math Function1/1 -> Sum of Elements1/1
  Unit Delay3/1 -> Math Function1/1
  Sum of Elements1/1 -> Sqrt2/1
  u_cap_dq1/1 -> FRT Slow Down/1(U), Unit Delay3/1
  Sqrt2/1 -> Switch/2, Switch1/2
  PF-Statik/1 -> Sum4/2
  P Filter Init/1(dP) -> Sum5/1
  [Ta] -> Divide3/1
  Sum8/1 -> P Filter Init/2(dP0), Scope2/1, Sum5/2, Scope1/1
  sp_VSM/1 -> Bus Selector3/1, Bus Selector2/1
  Bus Selector3/1 -> Selector1/1  "<sp_PQ>"
  Integrator (Inertia)/1(omega [pu]) -> Sum3/2, omega0/1
  [Enable] -> Integrator (Inertia)/Enable
  Forward Damping/1 -> Sum1/2
  Saturation1/1 -> Mux/1, [E]
  omega0/1 -> [omega], Integrator (Angle)/2(omega)
  [Enable] -> Integrator (Angle)/1(Reset)
  [E0] -> Saturation/1
  Unit Delay2/1 -> Sum2/1
  [Tu] -> Q(U)-PI-Regler/1(Tau)
  [phi] -> Bus Creator3/4  "phi"
  Bus Selector13/6 -> [TPinit]  "<TPinit>"
  [E] -> Bus Creator3/5  "E"
  [ku] -> QU-Statik/2
  Sum2/1 -> Q(U)-PI-Regler/2(E)
  Data Type Conversion/1 -> [Enable]
  Unit Delay1/1 -> Subsystem/1(first_run)
  Constant2/1 -> Unit Delay1/1
  u_inv_dq/1 -> Subsystem/2(u_dq)
  [Enable] -> Detect Increase/1
  Param/1 -> Bus Selector13/1
  Bus Selector13/1 -> [Ta]  "<Ta>"
  Bus Selector13/2 -> [kpf]  "<kpf>"
  Bus Selector13/3 -> [kdf]  "<kdf>"
  Bus Selector13/4 -> [ku]  "<ku>"
  Bus Selector13/5 -> [Tu]  "<Tu>"
  [Enable] -> Logical Operator1/1
  Logical Operator1/1 -> P Filter Init/Enable
  Compare To Zero1/1 -> Logical Operator1/2
  [TPinit] -> Compare To Zero1/1, P Filter Init/1(Tau)
  Sum5/1 -> [d_P], Sum4/1
  Detect Increase/1 -> Subsystem/Enable
  Subsystem/2(u_ang) -> [phi0]
  Constant/1 -> Mux/2
  Mux/1 -> sp_u_inv_dq/1
  [pll_om] -> Integrator (Inertia)/2(omega0 [pu])
  Divide3/1 -> Integrator (Inertia)/1(dPTa)
  Bus Selector11/1 -> Selector3/1  "<vdq>"
  PQ_meas/1 -> Selector2/1
  [sp_VSM] -> Bus Creator3/6, Scope/1  "sp_VSM"
  omega3/1 -> Bus Creator3/3  "mdelta_f"
  omega2/1 -> Bus Creator3/2  "f"
  [d_omega] -> omega3/1
  omega1/1 -> [d_omega], Forward Damping/2
  [omega] -> omega2/1
  Bus Creator3/1 -> VSMdiag/1
  PLL/1 -> Bus Selector11/1
  Bus Selector2/1 -> 1/f1/1, Bus Creator/1  "<sp_f>"
  Sum3/1 -> omega1/1, PF-Statik/2
  Sum4/1 -> Divide3/2
  Sum1/1 -> phi_rad/1, [phi]  "Phi [rad]"
  [Enable] -> Bus Creator3/7  "VSM_enable"
  Selector3/1 -> Subsystem/3(u_dq_pll)
  Integrator (Angle)/1(phi) -> Sum1/1
  Bus Selector11/3 -> 1/f3/1  "<f>"
  1/f3/1 -> [pll_om]
  [kdf] -> Forward Damping/1
  [kpf] -> PF-Statik/1
  "PQ_meas "/1 -> Selector5/1
  Bus Selector1/2 -> Selector6/1  "<sp_PQ>"
  "sp_VSM "/1 -> Bus Selector1/1
  Sum6/1 -> [d_Q], QU-Statik/1
  Selector2/1 -> Sum8/1, Enabled Subsystem1/1(P)
  Mux1/1 -> Bus Creator3/1  "delta_PQ"
  [d_P] -> Mux1/1
  [d_Q] -> Mux1/2
  1/f1/1 -> Sum3/1
  Selector6/1 -> Sum6/1, Mux2/2
  Selector5/1 -> Sum6/2
  Bus Selector11/2 -> Subsystem/4(phi_pll)  "<phi>"
  [Enable] -> Q(U)-PI-Regler/Enable

== system VSM_specComp_DC_22a/VSM_3/VSM1/VSM/CONTROL/Virtual Circuit mit R und L/Current Predictor ==
  u : Inport
  Delay : Delay  DelayLength=1  InitialCondition=0
  Sum : Sum  Inputs=|-+
  Sum1 : Sum  Inputs=|++
  y : Outport
  wires:
  Sum1/1 -> y/1
  Sum/1 -> Sum1/1
  Delay/1 -> Sum/1
  u/1 -> Delay/1, Sum1/2, Sum/2

== system VSM_specComp_DC_22a/VSM_3/VSM1/VSM/CONTROL/Virtual Circuit mit R und L/PT1 ==
  U : Inport  SampleTime=Ts
  tau : Inport  Port=2  SampleTime=Ts
  Reset : Inport  Port=3  SampleTime=Ts
  Phi : Inport  Port=4
  Delay : Delay  DelayLength=1  InitialConditionSource=Input port  ExternalReset=Rising
      settings: InputPortMap=u0,r5,p4
  Divide : Product  Inputs=*/
  Gain : Gain  Gain=Ts
  Gain1 : Gain  Gain=K
  Saturation : Saturate  UpperLimit=inf  LowerLimit=Ts
  Sum : Sum  Inputs=|++
  Sum2 : Sum  Inputs=|+-
  Unit Delay2 : UnitDelay  InitialCondition=[0 0 0]  SampleTime=ControlSampleTime  HasFrameUpgradeWarning=on
  dq0->ab0 phi : FriedrichLibrary/Transformations/dq0->ab0 phi  SystemSampleTime=-1  VariantActivationTime=update diagram  Latency=0  AutoFrameSizeCalculation=off
  Y : Outport
  wires:
  dq0->ab0 phi/1 -> Delay/3
  Gain1/1 -> Y/1
  Sum2/1 -> Gain/1
  U/1 -> Sum2/1
  Gain/1 -> Divide/1
  Delay/1 -> Sum/2, Sum2/2
  tau/1 -> Saturation/1
  Divide/1 -> Sum/1
  Saturation/1 -> Divide/2
  Reset/1 -> Delay/2
  Sum/1 -> Delay/1, Unit Delay2/1, Gain1/1
  Unit Delay2/1 -> dq0->ab0 phi/1
  Phi/1 -> dq0->ab0 phi/2

== system VSM_specComp_DC_22a/VSM_3/VSM1/VSM/CONTROL/Virtual Circuit mit R und L/PT2 ==
  U : Inport  SampleTime=Ts
  tau : Inport  Port=2  SampleTime=Ts
  Reset : Inport  Port=3  SampleTime=Ts
  Phi : Inport  Port=4
  Delay : Delay  DelayLength=1  InitialConditionSource=Input port  ExternalReset=Rising
      settings: InputPortMap=u0,r5,p4
  Divide : Product  Inputs=*/
  Gain : Gain  Gain=Ts
  Gain1 : Gain  Gain=K
  Saturation : Saturate  UpperLimit=inf  LowerLimit=Ts
  Sum : Sum  Inputs=|++
  Sum2 : Sum  Inputs=|+-
  Unit Delay2 : UnitDelay  InitialCondition=[0 0 0]  SampleTime=ControlSampleTime  HasFrameUpgradeWarning=on
  dq0->ab0 phi1 : FriedrichLibrary/Transformations/dq0->ab0 phi  SystemSampleTime=-1  VariantActivationTime=update diagram  Latency=0  AutoFrameSizeCalculation=off
  Y : Outport
  wires:
  Phi/1 -> dq0->ab0 phi1/2
  Unit Delay2/1 -> dq0->ab0 phi1/1
  Sum/1 -> Gain1/1, Unit Delay2/1, Delay/1
  Reset/1 -> Delay/2
  Saturation/1 -> Divide/2
  Divide/1 -> Sum/1
  tau/1 -> Saturation/1
  Delay/1 -> Sum2/2, Sum/2
  Gain/1 -> Divide/1
  U/1 -> Sum2/1
  Sum2/1 -> Gain/1
  Gain1/1 -> Y/1
  dq0->ab0 phi1/1 -> Delay/3

== system VSM_specComp_DC_22a/VSM_3/VSM1/VSM/CONTROL/Virtual Circuit1/Current Predictor ==
  u : Inport
  Delay : Delay  DelayLength=1  InitialCondition=0
  Sum : Sum  Inputs=|-+
  Sum1 : Sum  Inputs=|++
  y : Outport
  wires:
  Sum1/1 -> y/1
  Sum/1 -> Sum1/1
  Delay/1 -> Sum/1
  u/1 -> Delay/1, Sum1/2, Sum/2

== system VSM_specComp_DC_22a/VSM_3/VSM1/VSM/CONTROL/Virtual Circuit1/PT1 ==
  U : Inport  SampleTime=Ts
  tau : Inport  Port=2  SampleTime=Ts
  Reset : Inport  Port=3  SampleTime=Ts
  Delay : Delay  DelayLength=1
  Divide : Product  Inputs=*/
  Gain : Gain  Gain=Ts
  Gain1 : Gain  Gain=K
  Saturation : Saturate  UpperLimit=inf  LowerLimit=Ts
  Sum : Sum  Inputs=|++
  Sum2 : Sum  Inputs=|+-
  Switch : Switch  Criteria=u2 > Threshold  SaturateOnIntegerOverflow=off  InputSameDT=off
  Y : Outport
  wires:
  Sum/1 -> Switch/3
  Switch/1 -> Delay/1, Gain1/1
  Gain1/1 -> Y/1
  Sum2/1 -> Gain/1
  U/1 -> Sum2/1, Switch/1
  Gain/1 -> Divide/1
  Delay/1 -> Sum/2, Sum2/2
  tau/1 -> Saturation/1
  Divide/1 -> Sum/1
  Saturation/1 -> Divide/2
  Reset/1 -> Switch/2

== system VSM_specComp_DC_22a/VSM_3/VSM1/VSM/CONTROL/Virtual Circuit1/PT2 ==
  U : Inport  SampleTime=Ts
  tau : Inport  Port=2  SampleTime=Ts
  Reset : Inport  Port=3  SampleTime=Ts
  Phi : Inport  Port=4
  Delay : Delay  DelayLength=1  InitialConditionSource=Input port  ExternalReset=Rising
      settings: InputPortMap=u0,r5,p4
  Divide : Product  Inputs=*/
  Gain : Gain  Gain=Ts
  Gain1 : Gain  Gain=K
  Saturation : Saturate  UpperLimit=inf  LowerLimit=Ts
  Sum : Sum  Inputs=|++
  Sum2 : Sum  Inputs=|+-
  Unit Delay2 : UnitDelay  InitialCondition=[0 0 0]  SampleTime=ControlSampleTime  HasFrameUpgradeWarning=on
  dq0->ab0 phi1 : FriedrichLibrary/Transformations/dq0->ab0 phi  SystemSampleTime=-1  VariantActivationTime=update diagram  Latency=0  AutoFrameSizeCalculation=off
  Y : Outport
  wires:
  Phi/1 -> dq0->ab0 phi1/2
  Unit Delay2/1 -> dq0->ab0 phi1/1
  Sum/1 -> Gain1/1, Unit Delay2/1, Delay/1
  Reset/1 -> Delay/2
  Saturation/1 -> Divide/2
  Divide/1 -> Sum/1
  tau/1 -> Saturation/1
  Delay/1 -> Sum2/2, Sum/2
  Gain/1 -> Divide/1
  U/1 -> Sum2/1
  Sum2/1 -> Gain/1
  Gain1/1 -> Y/1
  dq0->ab0 phi1/1 -> Delay/3

== system VSM_specComp_DC_22a/VSM_3/VSM1/VSM/CONTROL/i_dq_ctrl/PI ==
  di : Inport
  u0 : Inport  Port=2
  Enable : EnablePort  StatesWhenEnabling=reset
  Gain4 : Gain  Gain=Ki
  Gain5 : Gain  Gain=Kp
  Integrator (inertia) : DiscreteIntegrator  gainval=1  InitialConditionSource=external  InitialCondition=1  SampleTime=ControlSampleTime  ICPrevOutput=DiscIntNeverNeededParam  ICPrevScaledInput=DiscIntNeverNeededParam
  Product : Product
  Product1 : Product
  Step : Step  Time=8  Before=1  SampleTime=0
  Step1 : Step  Time=8.05+10  Before=1  After=0.1  SampleTime=0
  Sum2 : Sum  Inputs=++|
  u : Outport  VectorParamsAs1DForOutWhenUnconnected=off
  wires:
  Step1/1 -> Product1/1
  Step/1 -> Product/1
  Product/1 -> Sum2/1
  Product1/1 -> Integrator (inertia)/1
  Gain4/1 -> Product1/2
  Gain5/1 -> Product/2
  Integrator (inertia)/1 -> Sum2/2
  di/1 -> Gain5/1, Gain4/1
  Sum2/1 -> u/1
  u0/1 -> Integrator (inertia)/2

== system VSM_specComp_DC_22a/VSM_3/VSM1/VSM/MANAGEMENT/Subsystem1/Subsystem ==
  note: zweiter Faktor bei clearing für richtiges Q
      |
      | bei Eintritt mit Halten aber fester Grenze
      |
      | bis jetzt über Zeit abgeschaltet bei clearing ohne Halten
  i_inv : Inport
  PQ_out : Inport  Port=2
  iabs : Inport  Port=3
  U_cap : Inport  Port=4
  PQ_pre : Inport  Port=5
  i abs_pre : Inport  Port=6
  Enable : EnablePort
  Abs : Abs  SaturateOnIntegerOverflow=off
  Add : Sum  Inputs=+-
  Demux : Demux  Commented=on  Outputs=3
  Discrete Derivative1 : simulink/Discrete/Discrete Derivative  Commented=on  gainval=1.0  ICPrevScaledInput=0.0  OutMin=[]  OutMax=[]  OutDataType=fixdt(1, 16)  OutScaling=2^-10  DoSatur=off
  Discrete Derivative2 : simulink/Discrete/Discrete Derivative  gainval=1.0  ICPrevScaledInput=0.0  OutMin=[]  OutMax=[]  OutDataType=fixdt(1, 16)  OutScaling=2^-10  DoSatur=off
  Divide : Product  Inputs=*/
  Divide1 : Product  Commented=on  Inputs=*/
  MATLAB Function1 : MATLAB Function  TreatAsAtomicUnit=on  SystemSampleTime=ControlSampleTime
  MATLAB Function2 : MATLAB Function  Commented=on  TreatAsAtomicUnit=on  SystemSampleTime=ControlSampleTime
  Mean : spsMeanLib/Mean  Freq=2000/2  Vinit=0  Ts=0
  Mux : Mux  Commented=on  Inputs=3
  Rate Transition : RateTransition  Commented=on  OutPortSampleTime=ControlSampleTime
  Scope : Scope  NumInputPorts=2
  Selector1 : Selector  Commented=on  InputPortWidth=3  IndexOptions=Index vector (dialog)  Indices=2  OutputSizes=1
  Selector2 : Selector  InputPortWidth=3  IndexOptions=Index vector (dialog)  Indices=1  OutputSizes=1
  T->ControlSampleTime : Subsystem  Commented=on  TreatAsAtomicUnit=on  SystemSampleTime=ControlSampleTime
  Transfer Fcn : TransferFcn  Commented=on  Denominator=[0.0001 1]
  Transport Delay : TransportDelay  DelayTime=0.002
  i_sp : Outport
  CC : Outport  Port=2
  wires:
  Mean/1 -> MATLAB Function1/4(der)
  Discrete Derivative2/1 -> Abs/1
  Abs/1 -> Mean/1
  Divide1/1 -> Discrete Derivative1/1
  Selector1/1 -> Divide1/1
  i_inv/1 -> MATLAB Function1/1(i_inv), T->ControlSampleTime/1(In1), Selector2/1, Selector1/1
  Add/1 -> MATLAB Function1/8(u_diff), Scope/2
  Transport Delay/1 -> Add/2
  i abs_pre/1 -> MATLAB Function1/7(i_abs_pre)
  PQ_pre/1 -> MATLAB Function1/6(i_pq_pre)
  Divide/1 -> Discrete Derivative2/1
  Selector2/1 -> Divide/1
  MATLAB Function1/2(CC) -> CC/1
  MATLAB Function1/1(i_sp) -> i_sp/1, Scope/1
  Rate Transition/1 -> Mux/2
  Demux/3 -> Mux/3
  Demux/1 -> Mux/1
  Transfer Fcn/1 -> Rate Transition/1
  Demux/2 -> Transfer Fcn/1
  U_cap/1 -> MATLAB Function1/5(U_cap), Divide/2, Divide1/2, Transport Delay/1, Add/1
  T->ControlSampleTime/1(Out1) -> Demux/1
  iabs/1 -> MATLAB Function1/3(i_abs)
  PQ_out/1 -> MATLAB Function1/2(PQ_out)

== system VSM_specComp_DC_22a/VSM_3/VSM1/VSM/MANAGEMENT/Subsystem1/Subsystem1 ==
  In1 : Inport
  In2 : Inport  Port=2
  Enable : EnablePort
  i_pq_pre : Outport
  i_abs_pre : Outport  Port=2
  wires:
  In2/1 -> i_abs_pre/1
  In1/1 -> i_pq_pre/1

== system VSM_specComp_DC_22a/VSM_3/VSM1/VSM/MANAGEMENT/sp_VSM/E(PQ) ==
  E : Inport
  cmd : Inport  Port=2
  sp_PQ : Inport  Port=3
  Abs : Abs  SaturateOnIntegerOverflow=off
  Add : Sum
  Add1 : Sum  Inputs=--
  Add2 : Sum  Inputs=+++
  Bus Selector : BusSelector  OutputSignals=Param.VC.R1,Param.VC.R1t,Param.VC.L1,Param.VC.L1t,Param.VSM.ku
  Bus Selector1 : BusSelector  OutputSignals=Param.VSM.sp_E_comp
  Constant : Constant
  Demux : Demux  Outputs=2
  Display{,1..4} (5 alike) : Display
  Divide : Product  Inputs=/*
  Product : Product
  Product1 : Product
  Real-Imag to Complex : RealImagToComplex
  Real-Imag to Complex1 : RealImagToComplex
  Switch : Switch  Criteria=u2 ~= 0  SaturateOnIntegerOverflow=off  InputSameDT=off
  "cmd " : InportShadow  Port=2
  sp_E : Outport  VectorParamsAs1DForOutWhenUnconnected=off
  wires:
  Constant/1 -> Add2/1, Divide/1
  Product1/1 -> Add2/3
  Bus Selector/5 -> Product1/2  "<ku>"
  Bus Selector1/1 -> Switch/2  "<sp_E_comp>"
  "cmd "/1 -> Bus Selector1/1
  Switch/1 -> sp_E/1
  cmd/1 -> Bus Selector/1
  Bus Selector/1 -> Add/1  "<R1>"
  Bus Selector/2 -> Add/2  "<R1t>"
  Bus Selector/3 -> Add1/1  "<L1>"
  Bus Selector/4 -> Add1/2  "<L1t>"
  Add/1 -> Real-Imag to Complex/1
  Add1/1 -> Real-Imag to Complex/2
  E/1 -> Switch/3
  sp_PQ/1 -> Demux/1
  Demux/1 -> Real-Imag to Complex1/1
  Demux/2 -> Real-Imag to Complex1/2, Product1/1
  Real-Imag to Complex1/1 -> Divide/2
  Divide/1 -> Product/1, Display/1  "current"
  Real-Imag to Complex/1 -> Product/2, Display1/1  "impedance"
  Product/1 -> Add2/2, Display2/1  "voltage"
  Abs/1 -> Switch/1, Display4/1
  Add2/1 -> Abs/1, Display3/1
